simulink model "bsm1_ss"  (Simulink 8.0)
settings: Solver=ode15s  SolverMode=SingleTasking  StartTime=0.0  StopTime=200  FixedStep=0.01  RelTol=1e-5  AbsTol=1e-8
values from neighbouring files (symbols this model uses):
  ACTIVATE = [ 0 ]    [init_bsm1.m]
  carb1 = 0    [reginit_bsm1.m]    (also in reginit_bsm1_2.m)
  carb2 = 0    [reginit_bsm1.m]    (also in reginit_bsm1_2.m)
  carb3 = 0    [reginit_bsm1.m]    (also in reginit_bsm1_2.m)
  carb4 = 0    [reginit_bsm1.m]    (also in reginit_bsm1_2.m)
  carb5 = 0    [reginit_bsm1.m]    (also in reginit_bsm1_2.m)
  KLa1 = 2    [reginit_bsm1.m]    (also in reginit_bsm1_2.m)
  KLa2 = 2    [reginit_bsm1.m]    (also in reginit_bsm1_2.m)
  KLa3 = 240    [reginit_bsm1.m]    (also in reginit_bsm1_2.m)
  KLa4 = 240    [reginit_bsm1.m]    (also in reginit_bsm1_2.m)
  KLa5 = 240    [reginit_bsm1.m]    (also in reginit_bsm1_2.m)
  PAR2 = PAR1    [mcsim.m]
  PAR3 = PAR1    [mcsim.m]
  PAR4 = PAR1    [mcsim.m]
  PAR5 = PAR1    [mcsim.m]
  T = 0.0001    [hyddelayinit_bsm1.m]
  TEMPMODEL = [ 0 ]    [init_bsm1.m]
  XINITDELAY = [ S_I_ASin  S_S_ASin  X_I_ASin  X_S_ASin  X_BH_ASin  X_BA1_ASin  X_P_ASin  S_O_ASin  S_NO3_ASin  S_NH_ASin  S_ND_ASin  X_ND_ASin  S_ALK_ASin TSS_ASin Q_ASin T_ASin    S_NO2_ASin S_NO_ASin S_N2O_ASin S_N2_ASin X_BA2_ASin    S_D1_ASin S_D2_ASin S_D3_ASin X_D4_ASin X_D5_ASin ]    [hyddelayinit_bsm1.m]
undefined symbols (not defined in the file or in its folder): PAR1, Qintr, Qr, Qw, SOSAT1, SOSAT2, SOSAT3, SOSAT4, SOSAT5, VOL1, VOL2, VOL3, VOL4, VOL5, XINIT1, XINIT2, XINIT3, XINIT4, XINIT5
settings Model: Creator=ielulf  LastModifiedBy=lasn  ExtModeTrigMode=oneshot  ExtModeArmWhenConnect=off  ExtModeAutoUpdateStatusClock=off  BufferReuse=off
settings DataIOCC: InitialState=xFinal  LimitDataPoints=off  SignalLoggingSaveFormat=ModelDataLogs  SaveOutput=off  TimeSaveName=t  SignalLoggingName=sigsOut  OutputTimes=[0:(1/96):609]
settings OptimizationCC: BlockReduction=off  BooleanDataType=off  InlineInvariantSignals=on  OptimizeBlockIOStorage=off  BufferReuse=off  ExpressionFolding=off  LocalBlockOutputs=off  InitFltsAndDblsToZero=on
settings DebuggingCC: SaveWithParameterizedLinksMsg=none  SignalResolutionControl=TryResolveAllWithWarning  SolverPrmCheckMsg=none  InheritedTsInSrcMsg=none  MultiTaskDSMMsg=warning  MultiTaskCondExecSysMsg=none  FcnCallInpInsideContextMsg=UseLocalSettings  UnconnectedOutputMsg=none  StrictBusMsg=None
settings HardwareCC: TargetUnknown=on
settings RTWCC: TemplateMakefile=grt_unix.tmf  IncludeERTFirstTime=on
settings GRTTargetCC: TargetFcnLib=ansi_tfl_tmw.mat  CombineOutputUpdateFcns=off  GRTInterface=on

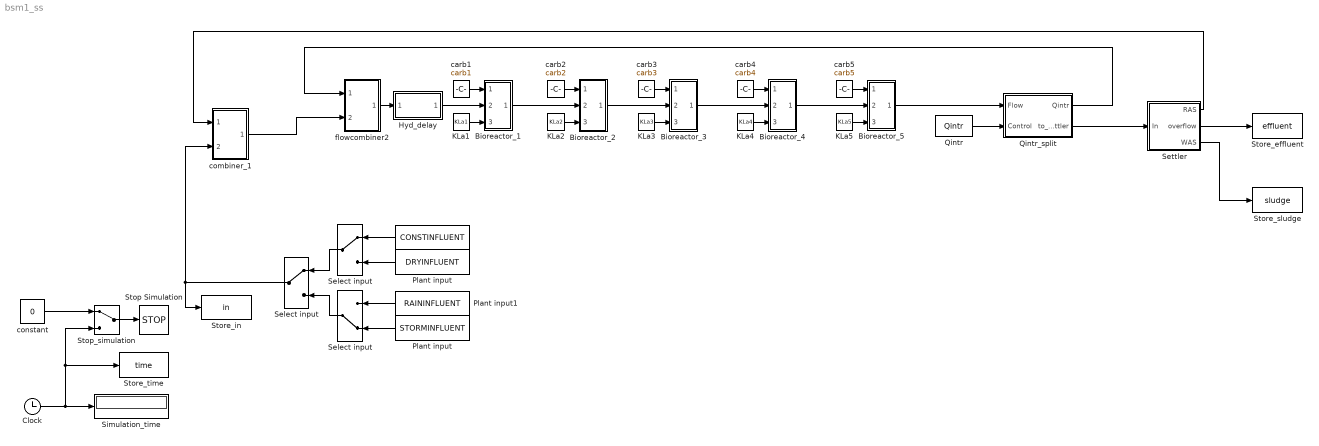
== system bsm1_ss ==
  " " : FromWorkspace  VariableName=CONSTINFLUENT  OutputAfterFinalValue=Holding final value
  " Select input" : ManualSwitch
  " constant" : Constant  Value=0
  Bioreactor_1 : Subsystem
  Bioreactor_2 : Subsystem
  Bioreactor_3 : Subsystem
  Bioreactor_4 : Subsystem
  Bioreactor_5 : Subsystem
  Clock : Clock
  Hyd_delay : Subsystem
  KLa1 : Constant  Value=KLa1
  KLa2 : Constant  Value=KLa2
  KLa3 : Constant  Value=KLa3
  KLa4 : Constant  Value=KLa4
  KLa5 : Constant  Value=KLa5
  Plant input : FromWorkspace  VariableName=DRYINFLUENT  OutputAfterFinalValue=Holding final value
  "Plant input " : FromWorkspace  VariableName=STORMINFLUENT  OutputAfterFinalValue=Holding final value
  Plant input1 : FromWorkspace  VariableName=RAININFLUENT  OutputAfterFinalValue=Holding final value
  Qintr : Constant  Value=Qintr
  Qintr_split : Subsystem
  Select input : ManualSwitch
  "Select input " : ManualSwitch  CurrentSetting=0
  Settler : Subsystem
  Simulation_time : Display
  Stop Simulation : Stop
  Stop_simulation : ManualSwitch
  Store_effluent : ToWorkspace  VariableName=effluent
  Store_in : ToWorkspace  VariableName=in  SampleTime=-1
  Store_sludge : ToWorkspace  VariableName=sludge
  Store_time : ToWorkspace  VariableName=time
  carb1 : Constant  Value=carb1
  carb2 : Constant  Value=carb2
  carb3 : Constant  Value=carb3
  carb4 : Constant  Value=carb4
  carb5 : Constant  Value=carb5
  combiner_1 : Subsystem
  flowcombiner2 : Subsystem
  wires:
  Clock/1 -> Simulation_time/1, Stop_simulation/2, Store_time/1
  Stop_simulation/1 -> Stop Simulation/1
  " constant"/1 -> Stop_simulation/1
  flowcombiner2/1(Out) -> Hyd_delay/1(Input)
  Qintr/1 -> Qintr_split/2(Control)
  Bioreactor_5/1(out) -> Qintr_split/1(Flow)
  Hyd_delay/1(Output) -> Bioreactor_1/2(in)
  KLa1/1 -> Bioreactor_1/3(KLa)
  Bioreactor_1/1(out) -> Bioreactor_2/2(in)
  KLa2/1 -> Bioreactor_2/3(KLa)
  Bioreactor_2/1(out) -> Bioreactor_3/2(in)
  KLa3/1 -> Bioreactor_3/3(KLa)
  Bioreactor_3/1(out) -> Bioreactor_4/2(in)
  KLa4/1 -> Bioreactor_4/3(KLa)
  Bioreactor_4/1(out) -> Bioreactor_5/2(in)
  KLa5/1 -> Bioreactor_5/3(KLa)
  carb1/1 -> Bioreactor_1/1(carb)
  carb2/1 -> Bioreactor_2/1(carb)
  carb3/1 -> Bioreactor_3/1(carb)
  carb4/1 -> Bioreactor_4/1(carb)
  carb5/1 -> Bioreactor_5/1(carb)
  combiner_1/1(Out) -> flowcombiner2/2(Qin)
  Qintr_split/1(Qintr) -> flowcombiner2/1(Qintr)
  Qintr_split/2(to_settler) -> Settler/1(In)
  Settler/1(RAS) -> combiner_1/1(In1)
  Settler/2(overflow) -> Store_effluent/1
  Settler/3(WAS) -> Store_sludge/1
  Plant input/1 -> Select input/2
  " "/1 -> Select input/1
  Plant input1/1 -> "Select input "/1
  "Plant input "/1 -> "Select input "/2
  Select input/1 -> " Select input"/1
  "Select input "/1 -> " Select input"/2
  " Select input"/1 -> combiner_1/2(In2), Store_in/1

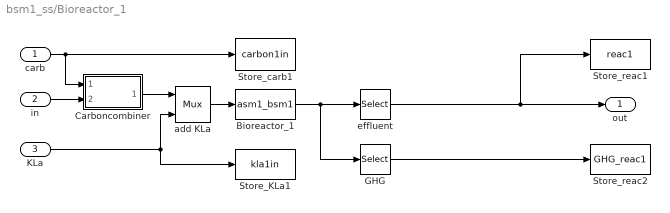
== system bsm1_ss/Bioreactor_1 ==
  carb : Inport
  in : Inport  Port=2
  KLa : Inport  Port=3
  Bioreactor_1 : S-Function  FunctionName=asm1_bsm1  Parameters=XINIT1,PAR1,VOL1,SOSAT1,TEMPMODEL,ACTIVATE  EnableBusSupport=off
  Carboncombiner : Subsystem
  GHG : Selector  InputPortWidth=29  IndexOptions=Index vector (dialog)  Indices=[27:29]  OutputSizes=1
  Store_KLa1 : ToWorkspace  VariableName=kla1in  SampleTime=-1
  Store_carb1 : ToWorkspace  VariableName=carbon1in  SampleTime=-1
  Store_reac1 : ToWorkspace  VariableName=reac1  SampleTime=-1
  Store_reac2 : ToWorkspace  VariableName=GHG_reac1  SampleTime=-1
  add KLa : Mux  Inputs=2
  effluent : Selector  InputPortWidth=29  IndexOptions=Index vector (dialog)  Indices=[1:26]  OutputSizes=1
  out : Outport
  wires:
  KLa/1 -> Store_KLa1/1, add KLa/2
  in/1 -> Carboncombiner/2(Input)
  carb/1 -> Carboncombiner/1(C_flow), Store_carb1/1
  Carboncombiner/1(Output) -> add KLa/1
  add KLa/1 -> Bioreactor_1/1
  Bioreactor_1/1 -> effluent/1, GHG/1
  effluent/1 -> out/1, Store_reac1/1
  GHG/1 -> Store_reac2/1

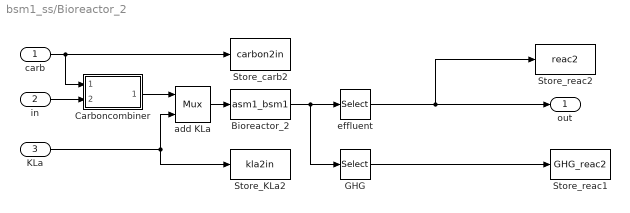
== system bsm1_ss/Bioreactor_2 ==
  carb : Inport
  in : Inport  Port=2
  KLa : Inport  Port=3
  Bioreactor_2 : S-Function  FunctionName=asm1_bsm1  Parameters=XINIT2,PAR2,VOL2,SOSAT2,TEMPMODEL,ACTIVATE  EnableBusSupport=off
  Carboncombiner : Subsystem
  GHG : Selector  InputPortWidth=29  IndexOptions=Index vector (dialog)  Indices=[27:29]  OutputSizes=1
  Store_KLa2 : ToWorkspace  VariableName=kla2in  SampleTime=-1
  Store_carb2 : ToWorkspace  VariableName=carbon2in  SampleTime=-1
  Store_reac1 : ToWorkspace  VariableName=GHG_reac2  SampleTime=-1
  Store_reac2 : ToWorkspace  VariableName=reac2  SampleTime=-1
  add KLa : Mux  Inputs=2
  effluent : Selector  InputPortWidth=29  IndexOptions=Index vector (dialog)  Indices=[1:26]  OutputSizes=1
  out : Outport
  wires:
  KLa/1 -> Store_KLa2/1, add KLa/2
  in/1 -> Carboncombiner/2(Input)
  carb/1 -> Store_carb2/1, Carboncombiner/1(C_flow)
  Carboncombiner/1(Output) -> add KLa/1
  add KLa/1 -> Bioreactor_2/1
  Bioreactor_2/1 -> GHG/1, effluent/1
  effluent/1 -> out/1, Store_reac2/1
  GHG/1 -> Store_reac1/1

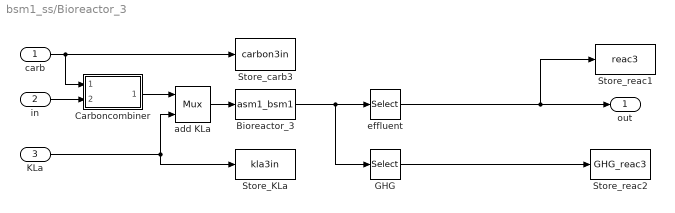
== system bsm1_ss/Bioreactor_3 ==
  carb : Inport
  in : Inport  Port=2
  KLa : Inport  Port=3
  Bioreactor_3 : S-Function  FunctionName=asm1_bsm1  Parameters=XINIT3,PAR3,VOL3,SOSAT3,TEMPMODEL,ACTIVATE  EnableBusSupport=off
  Carboncombiner : Subsystem
  GHG : Selector  InputPortWidth=29  IndexOptions=Index vector (dialog)  Indices=[27:29]  OutputSizes=1
  Store_KLa : ToWorkspace  VariableName=kla3in  SampleTime=-1
  Store_carb3 : ToWorkspace  VariableName=carbon3in  SampleTime=-1
  Store_reac1 : ToWorkspace  VariableName=reac3  SampleTime=-1
  Store_reac2 : ToWorkspace  VariableName=GHG_reac3  SampleTime=-1
  add KLa : Mux  Inputs=2
  effluent : Selector  InputPortWidth=29  IndexOptions=Index vector (dialog)  Indices=[1:26]  OutputSizes=1
  out : Outport
  wires:
  KLa/1 -> Store_KLa/1, add KLa/2
  in/1 -> Carboncombiner/2(Input)
  carb/1 -> Store_carb3/1, Carboncombiner/1(C_flow)
  Carboncombiner/1(Output) -> add KLa/1
  add KLa/1 -> Bioreactor_3/1
  Bioreactor_3/1 -> effluent/1, GHG/1
  effluent/1 -> out/1, Store_reac1/1
  GHG/1 -> Store_reac2/1

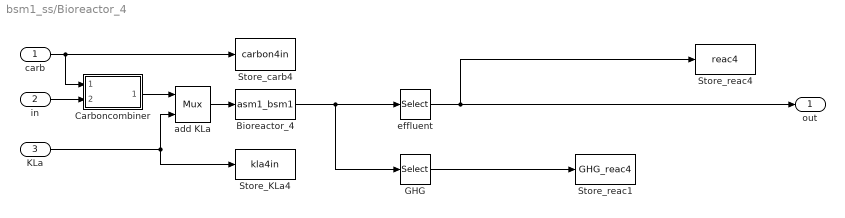
== system bsm1_ss/Bioreactor_4 ==
  carb : Inport
  in : Inport  Port=2
  KLa : Inport  Port=3
  Bioreactor_4 : S-Function  FunctionName=asm1_bsm1  Parameters=XINIT4,PAR4,VOL4,SOSAT4,TEMPMODEL,ACTIVATE  EnableBusSupport=off
  Carboncombiner : Subsystem
  GHG : Selector  InputPortWidth=29  IndexOptions=Index vector (dialog)  Indices=[27:29]  OutputSizes=1
  Store_KLa4 : ToWorkspace  VariableName=kla4in  SampleTime=-1
  Store_carb4 : ToWorkspace  VariableName=carbon4in  SampleTime=-1
  Store_reac1 : ToWorkspace  VariableName=GHG_reac4  SampleTime=-1
  Store_reac4 : ToWorkspace  VariableName=reac4  SampleTime=-1
  add KLa : Mux  Inputs=2
  effluent : Selector  InputPortWidth=29  IndexOptions=Index vector (dialog)  Indices=[1:26]  OutputSizes=1
  out : Outport
  wires:
  KLa/1 -> Store_KLa4/1, add KLa/2
  in/1 -> Carboncombiner/2(Input)
  carb/1 -> Store_carb4/1, Carboncombiner/1(C_flow)
  Carboncombiner/1(Output) -> add KLa/1
  add KLa/1 -> Bioreactor_4/1
  Bioreactor_4/1 -> GHG/1, effluent/1
  effluent/1 -> out/1, Store_reac4/1
  GHG/1 -> Store_reac1/1

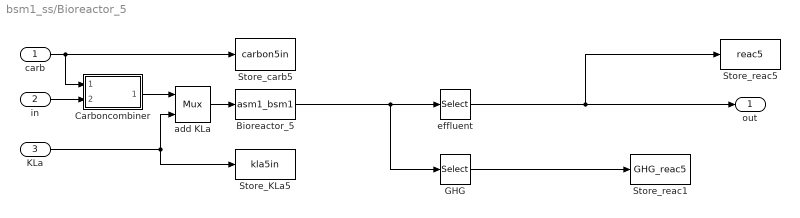
== system bsm1_ss/Bioreactor_5 ==
  carb : Inport
  in : Inport  Port=2
  KLa : Inport  Port=3
  Bioreactor_5 : S-Function  FunctionName=asm1_bsm1  Parameters=XINIT5,PAR5,VOL5,SOSAT5,TEMPMODEL,ACTIVATE  EnableBusSupport=off
  Carboncombiner : Subsystem
  GHG : Selector  InputPortWidth=29  IndexOptions=Index vector (dialog)  Indices=[27:29]  OutputSizes=1
  Store_KLa5 : ToWorkspace  VariableName=kla5in  SampleTime=-1
  Store_carb5 : ToWorkspace  VariableName=carbon5in  SampleTime=-1
  Store_reac1 : ToWorkspace  VariableName=GHG_reac5  SampleTime=-1
  Store_reac5 : ToWorkspace  VariableName=reac5  SampleTime=-1
  add KLa : Mux  Inputs=2
  effluent : Selector  InputPortWidth=29  IndexOptions=Index vector (dialog)  Indices=[1:26]  OutputSizes=1
  out : Outport
  wires:
  KLa/1 -> Store_KLa5/1, add KLa/2
  in/1 -> Carboncombiner/2(Input)
  carb/1 -> Store_carb5/1, Carboncombiner/1(C_flow)
  Carboncombiner/1(Output) -> add KLa/1
  add KLa/1 -> Bioreactor_5/1
  Bioreactor_5/1 -> GHG/1, effluent/1
  effluent/1 -> out/1, Store_reac5/1
  GHG/1 -> Store_reac1/1

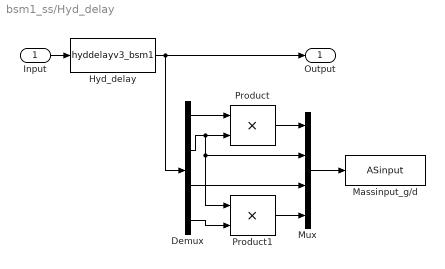
== system bsm1_ss/Hyd_delay ==
  Input : Inport
  Demux : Demux  Outputs=[14,1,1,10]
  Hyd_delay : S-Function  FunctionName=hyddelayv3_bsm1  Parameters=XINITDELAY,PAR1,T  EnableBusSupport=off
  Massinput_g/d : ToWorkspace  VariableName=ASinput  SampleTime=-1
  Mux : Mux
  Product : Product  SaturateOnIntegerOverflow=on  OutDataTypeStr=Inherit: Same as first input
  Product1 : Product  SaturateOnIntegerOverflow=on  OutDataTypeStr=Inherit: Same as first input
  Output : Outport
  wires:
  Mux/1 -> Massinput_g/d/1
  Product/1 -> Mux/1
  Demux/1 -> Product/1
  Hyd_delay/1 -> Output/1, Demux/1
  Input/1 -> Hyd_delay/1
  Demux/2 -> Product/2, Mux/2, Product1/1
  Demux/3 -> Mux/3
  Product1/1 -> Mux/4
  Demux/4 -> Product1/2

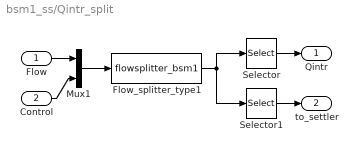
== system bsm1_ss/Qintr_split ==
  Flow : Inport
  Control : Inport  Port=2
  Flow_splitter_type1 : S-Function  FunctionName=flowsplitter_bsm1  Parameters=Qintrtype  EnableBusSupport=off
  Mux1 : Mux  Inputs=2
  Selector : Selector  InputPortWidth=52  IndexOptions=Index vector (dialog)  Indices=[1:26]  OutputSizes=1
  Selector1 : Selector  InputPortWidth=52  IndexOptions=Index vector (dialog)  Indices=[27:52]  OutputSizes=1
  Qintr : Outport
  to_settler : Outport  Port=2
  wires:
  Selector1/1 -> to_settler/1
  Control/1 -> Mux1/2
  Flow/1 -> Mux1/1
  Selector/1 -> Qintr/1
  Mux1/1 -> Flow_splitter_type1/1
  Flow_splitter_type1/1 -> Selector1/1, Selector/1

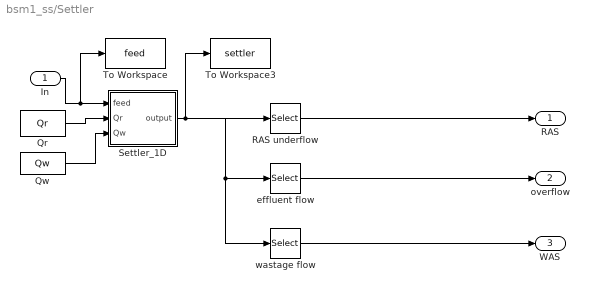
== system bsm1_ss/Settler ==
  In : Inport
  Qr : Constant  Value=Qr
  Qw : Constant  Value=Qw
  RAS underflow : Selector  InputPortWidth=253  IndexOptions=Index vector (dialog)  Indices=[226 227 228 229 230 231 232 233 234 235 236 237 238 239 252 240 241 242 243 244 245 246 247 248 249 250]  OutputSizes=1
  Settler_1D : Subsystem
  To Workspace : ToWorkspace  VariableName=feed
  To Workspace3 : ToWorkspace  VariableName=settler
  effluent flow : Selector  InputPortWidth=253  IndexOptions=Index vector (dialog)  Indices=[1:14, 251, 15:25]  OutputSizes=1
  wastage flow : Selector  InputPortWidth=253  IndexOptions=Index vector (dialog)  Indices=[226:239, 253, 240:250]  OutputSizes=1
  RAS : Outport
  overflow : Outport  Port=2
  WAS : Outport  Port=3
  wires:
  In/1 -> To Workspace/1, Settler_1D/1(feed)
  Settler_1D/1(output) -> To Workspace3/1, RAS underflow/1, effluent flow/1, wastage flow/1
  wastage flow/1 -> WAS/1
  effluent flow/1 -> overflow/1
  RAS underflow/1 -> RAS/1
  Qr/1 -> Settler_1D/2(Qr)
  Qw/1 -> Settler_1D/3(Qw)

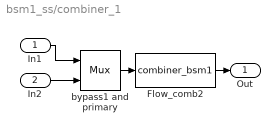
== system bsm1_ss/combiner_1 ==
  In1 : Inport
  In2 : Inport  Port=2
  Flow_comb2 : S-Function  FunctionName=combiner_bsm1  EnableBusSupport=off
  bypass1 and primary : Mux  Inputs=2
  Out : Outport
  wires:
  bypass1 and primary/1 -> Flow_comb2/1
  In1/1 -> bypass1 and primary/1
  Flow_comb2/1 -> Out/1
  In2/1 -> bypass1 and primary/2

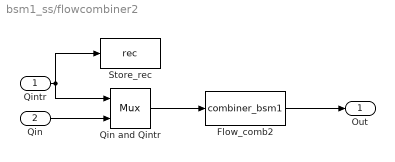
== system bsm1_ss/flowcombiner2 ==
  Qintr : Inport
  Qin : Inport  Port=2
  Flow_comb2 : S-Function  FunctionName=combiner_bsm1  EnableBusSupport=off
  Qin and Qintr : Mux  Inputs=2
  Store_rec : ToWorkspace  VariableName=rec
  Out : Outport
  wires:
  Qin and Qintr/1 -> Flow_comb2/1
  Qintr/1 -> Qin and Qintr/1, Store_rec/1
  Flow_comb2/1 -> Out/1
  Qin/1 -> Qin and Qintr/2

== system bsm1_ss/Bioreactor_1/Carboncombiner ==
  C_flow : Inport
  Input : Inport  Port=2
  Carboncombiner : S-Function  FunctionName=carboncombiner_bsm1  Parameters=CARBONSOURCECONC  EnableBusSupport=off
  Mux : Mux  Inputs=2
  Output : Outport
  wires:
  Input/1 -> Mux/2
  Carboncombiner/1 -> Output/1
  Mux/1 -> Carboncombiner/1
  C_flow/1 -> Mux/1

== system bsm1_ss/Bioreactor_2/Carboncombiner ==
  C_flow : Inport
  Input : Inport  Port=2
  Carboncombiner : S-Function  FunctionName=carboncombiner_bsm1  Parameters=CARBONSOURCECONC  EnableBusSupport=off
  Mux : Mux  Inputs=2
  Output : Outport
  wires:
  C_flow/1 -> Mux/1
  Mux/1 -> Carboncombiner/1
  Carboncombiner/1 -> Output/1
  Input/1 -> Mux/2

== system bsm1_ss/Bioreactor_3/Carboncombiner ==
  C_flow : Inport
  Input : Inport  Port=2
  Carboncombiner : S-Function  FunctionName=carboncombiner_bsm1  Parameters=CARBONSOURCECONC  EnableBusSupport=off
  Mux : Mux  Inputs=2
  Output : Outport
  wires:
  C_flow/1 -> Mux/1
  Mux/1 -> Carboncombiner/1
  Carboncombiner/1 -> Output/1
  Input/1 -> Mux/2

== system bsm1_ss/Bioreactor_4/Carboncombiner ==
  C_flow : Inport
  Input : Inport  Port=2
  Carboncombiner : S-Function  FunctionName=carboncombiner_bsm1  Parameters=CARBONSOURCECONC  EnableBusSupport=off
  Mux : Mux  Inputs=2
  Output : Outport
  wires:
  C_flow/1 -> Mux/1
  Mux/1 -> Carboncombiner/1
  Carboncombiner/1 -> Output/1
  Input/1 -> Mux/2

== system bsm1_ss/Bioreactor_5/Carboncombiner ==
  C_flow : Inport
  Input : Inport  Port=2
  Carboncombiner : S-Function  FunctionName=carboncombiner_bsm1  Parameters=CARBONSOURCECONC  EnableBusSupport=off
  Mux : Mux  Inputs=2
  Output : Outport
  wires:
  C_flow/1 -> Mux/1
  Mux/1 -> Carboncombiner/1
  Carboncombiner/1 -> Output/1
  Input/1 -> Mux/2

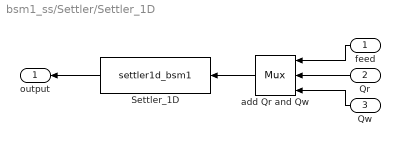
== system bsm1_ss/Settler/Settler_1D ==
  feed : Inport
  Qr : Inport  Port=2
  Qw : Inport  Port=3
  Settler_1D : S-Function  FunctionName=settler1d_bsm1  Parameters=SETTLERINIT,SETTLERPAR,DIM,LAYER,TEMPMODEL, ACTIVATE  EnableBusSupport=off
  add Qr and Qw : Mux  Inputs=3
  output : Outport
  wires:
  Settler_1D/1 -> output/1
  feed/1 -> add Qr and Qw/1
  Qw/1 -> add Qr and Qw/3
  Qr/1 -> add Qr and Qw/2
  add Qr and Qw/1 -> Settler_1D/1
